simulink model "assgn_3_model"  (R2021a)
settings: Solver=VariableStepAuto  StartTime=0.0  StopTime=10.0  RelTol=1e-3
undefined symbols (not defined in the file): A, B, x0
settings Model: Creator=vedan  LastModifiedBy=vedan

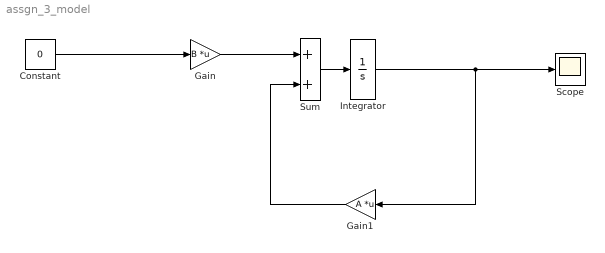
== system assgn_3_model ==
  Constant : Constant  Value=0
  Gain : Gain  Gain=B  Multiplication=Matrix(K*u)
  Gain1 : Gain  Gain=A  Multiplication=Matrix(K*u)
  Integrator : Integrator  InitialCondition=x0
  Scope : Scope
  Sum : Sum
  wires:
  Gain1/1 -> Sum/2
  Integrator/1 -> Gain1/1, Scope/1
  Constant/1 -> Gain/1
  Sum/1 -> Integrator/1
  Gain/1 -> Sum/1
